simulink model "IntegralBacksteppingDroneControl"  (R2023b)
settings: Solver=VariableStepAuto  StartTime=0.0  StopTime=10.0  RelTol=1e-3
libraries: simulink x1
settings Model: Creator=kevin  LastModifiedBy=kevin

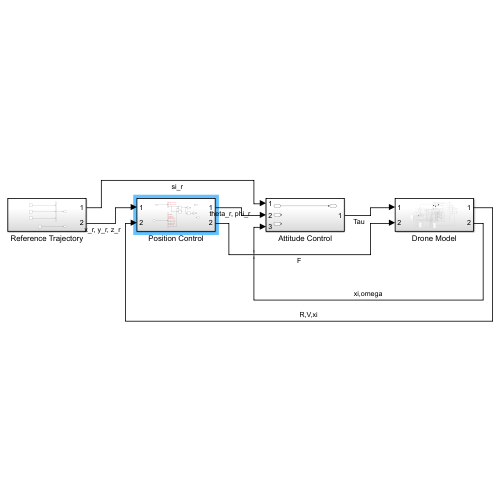
[thumbnail: Simulink's stored preview of the top-level diagram]
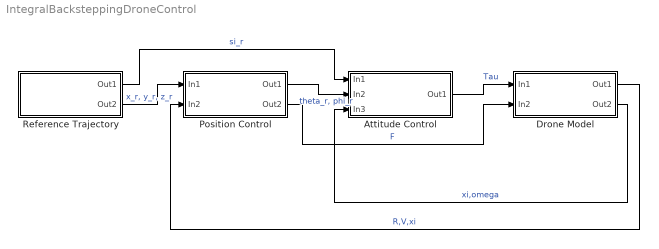
== system IntegralBacksteppingDroneControl ==
  Attitude Control : Subsystem
  Drone Model : Subsystem
  Position Control : Subsystem
  Reference Trajectory : Subsystem
  wires:
  Reference Trajectory/2(Out2) -> Position Control/1(In1)  "x_r, y_r, z_r"
  Reference Trajectory/1(Out1) -> Attitude Control/1(In1)  "si_r"
  Drone Model/1(Out1) -> Position Control/2(In2)  "R,V,xi"
  Drone Model/2(Out2) -> Attitude Control/3(In3)  "xi,omega"
  Position Control/1(Out1) -> Attitude Control/2(In2)  "theta_r, phi_r"
  Position Control/2(Out2) -> Drone Model/2(In2)  "F"
  Attitude Control/1(Out1) -> Drone Model/1(In1)  "Tau"

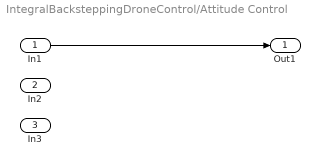
== system IntegralBacksteppingDroneControl/Attitude Control ==
  In1 : Inport
  In2 : Inport  Port=2
  In3 : Inport  Port=3
  Out1 : Outport
  wires:
  In1/1 -> Out1/1

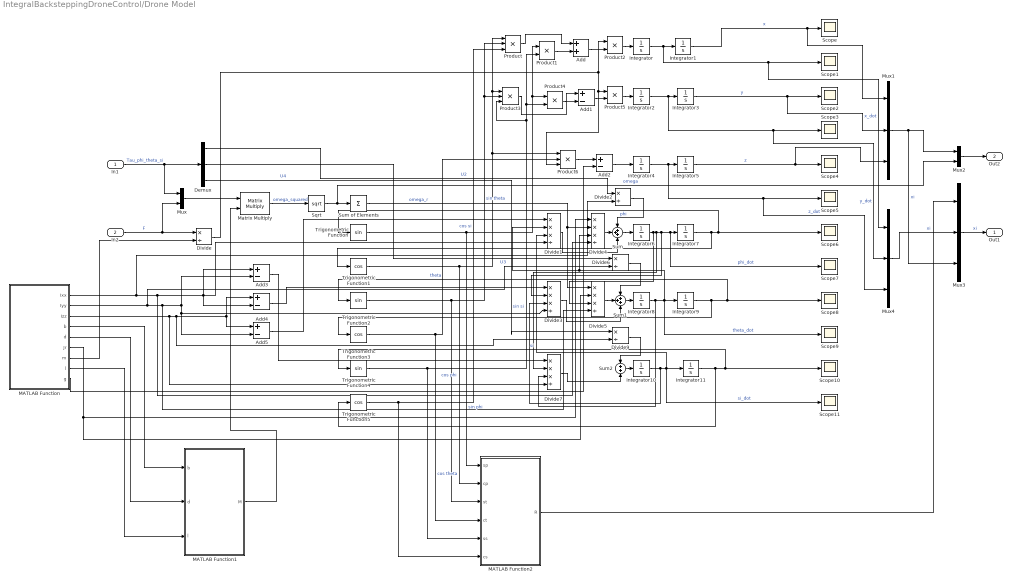
== system IntegralBacksteppingDroneControl/Drone Model ==
  In1 : Inport
  In2 : Inport  Port=2
  Add : Sum
  Add{1..5} (5 alike) : Sum  Inputs=+-
  Demux : Demux  Outputs=3
  Divide{,2,6,9} (4 alike) : Product  Inputs=*/
  Divide{1,3..5,7} (5 alike) : Product  Inputs=***/
  Integrator{,1..11} (12 alike) : Integrator
  MATLAB Function : MATLAB Function  TreatAsAtomicUnit=on
  MATLAB Function1 : MATLAB Function  TreatAsAtomicUnit=on
  MATLAB Function2 : MATLAB Function  TreatAsAtomicUnit=on
  Matrix Multiply : Product  Multiplication=Matrix(*)
  Mux : Mux  Inputs=2
  Mux1 : Mux  Inputs=3
  Mux2 : Mux  Inputs=2
  Mux3 : Mux  Inputs=3
  Mux4 : Mux  Inputs=3
  Product : Product  Inputs=3
  Product{1..2,4..5} (4 alike) : Product
  Product3 : Product  Inputs=3
  Product6 : Product  Inputs=3
  Scope{,1..11} (12 alike) : Scope
  Sqrt : Sqrt
  Sum : Sum  Inputs=+++
  Sum of Elements : Sum  Inputs=+
  Sum1 : Sum  Inputs=+++
  Sum2 : Sum
  Trigonometric Function : Trigonometry
  Trigonometric Function1 : Trigonometry  Operator=cos
  Trigonometric Function2 : Trigonometry
  Trigonometric Function3 : Trigonometry  Operator=cos
  Trigonometric Function4 : Trigonometry
  Trigonometric Function5 : Trigonometry  Operator=cos
  Out1 : Outport
  Out2 : Outport  Port=2
  wires:
  In1/1 -> Demux/1, Mux/1  "Tau_phi_theta_si"
  In2/1 -> Mux/2, Divide/1  "F"
  Demux/1 -> Divide2/1  "U2"
  Demux/2 -> Divide6/1  "U3"
  Demux/3 -> Divide9/1  "U4"
  Integrator1/1 -> Mux1/1, Scope/1  "x"
  Integrator/1 -> Mux4/1, Scope1/1, Integrator1/1  "x_dot"
  Integrator3/1 -> Mux1/2, Scope2/1  "y"
  Integrator2/1 -> Mux4/2, Scope3/1, Integrator3/1  "y_dot"
  Integrator5/1 -> Mux1/3, Scope4/1  "z"
  Integrator4/1 -> Mux4/3, Scope5/1, Integrator5/1  "z_dot"
  Integrator7/1 -> Trigonometric Function1/1, Trigonometric Function/1, Scope6/1  "phi"
  Integrator6/1 -> Divide5/3, Scope7/1, Integrator7/1, Divide3/2, Divide7/2  "phi_dot"
  Integrator9/1 -> Trigonometric Function3/1, Trigonometric Function2/1, Scope8/1  "theta"
  Integrator8/1 -> Divide7/3, Divide1/2, Divide4/3, Scope9/1, Integrator9/1  "theta_dot"
  Integrator11/1 -> Trigonometric Function5/1, Trigonometric Function4/1, Scope10/1  "si"
  Integrator10/1 -> Divide3/3, Divide1/3, Scope11/1, Integrator11/1  "si_dot"
  Trigonometric Function/1 -> MATLAB Function2/1(sp), Product1/1, Product4/1  "sin phi"
  Trigonometric Function1/1 -> MATLAB Function2/2(cp), Product3/1, Product/1, Product6/1  "cos phi"
  Trigonometric Function2/1 -> MATLAB Function2/3(st), Product3/2, Product/2  "sin theta"
  Trigonometric Function3/1 -> MATLAB Function2/4(ct), Product6/2  "cos theta"
  Trigonometric Function4/1 -> MATLAB Function2/5(ss), Product3/3, Product1/2, Product4/2  "sin si"
  Trigonometric Function5/1 -> MATLAB Function2/6(cs), Product/3  "cos si"
  Product/1 -> Add/1
  Product1/1 -> Add/2
  MATLAB Function/7(m) -> Divide/2
  Divide/1 -> Product2/1, Product6/3, Product5/1
  Product2/1 -> Integrator/1
  Add/1 -> Product2/2
  Product3/1 -> Add1/1
  Product4/1 -> Add1/2
  Product5/1 -> Integrator2/1
  Add1/1 -> Product5/2
  Product6/1 -> Add2/1
  MATLAB Function/9(g) -> Add2/2
  Add2/1 -> Integrator4/1
  MATLAB Function/4(b) -> MATLAB Function1/1(b)
  MATLAB Function/8(l) -> MATLAB Function1/3(l)
  MATLAB Function1/1(M) -> Matrix Multiply/2
  Mux/1 -> Matrix Multiply/1
  Matrix Multiply/1 -> Sqrt/1  "omega_squared"
  Sqrt/1 -> Mux2/2, Sum of Elements/1  "omega"
  Sum of Elements/1 -> Divide5/1, Divide4/2  "omega_r"
  Add3/1 -> Divide7/1
  Add4/1 -> Divide3/1
  Add5/1 -> Divide1/1
  Divide1/1 -> Sum/3
  MATLAB Function/5(d) -> MATLAB Function1/2(d)
  MATLAB Function/1(Ixx) -> Divide2/2, Divide4/4, Divide1/4, Add3/1, Add4/2
  Divide4/1 -> Sum/2
  Sum/1 -> Integrator6/1
  Divide2/1 -> Sum/1
  Sum1/1 -> Integrator8/1
  Divide5/1 -> Sum1/2
  Divide3/1 -> Sum1/3
  Divide6/1 -> Sum1/1
  MATLAB Function/6(Jr) -> Divide4/1, Divide5/2
  MATLAB Function/2(Iyy) -> Divide6/2, Divide5/4, Divide3/4, Add5/2, Add3/2
  Sum2/1 -> Integrator10/1
  Divide7/1 -> Sum2/2
  Divide9/1 -> Sum2/1
  MATLAB Function/3(Izz) -> Divide7/4, Divide9/2, Add5/1, Add4/1
  Mux1/1 -> Mux3/3, Mux2/1  "xi"
  Mux2/1 -> Out2/1
  MATLAB Function2/1(R) -> Mux3/1
  Mux3/1 -> Out1/1  "xi"
  Mux4/1 -> Mux3/2  "xi"

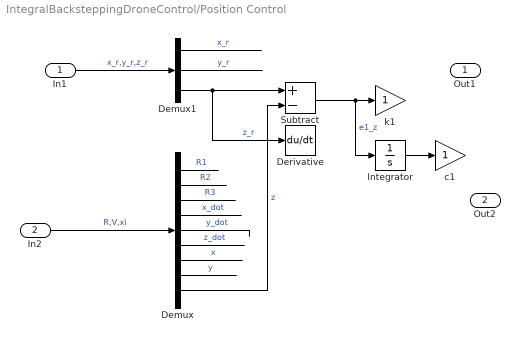
== system IntegralBacksteppingDroneControl/Position Control ==
  In1 : Inport
  In2 : Inport  Port=2
  Demux : Demux  Outputs=9
  Demux1 : Demux  Outputs=3
  Derivative : Derivative
  Integrator : Integrator
  Subtract : Sum  Inputs=+-
  c1 : Gain
  k1 : Gain
  Out1 : Outport
  Out2 : Outport  Port=2
  wires:
  In1/1 -> Demux1/1  "x_r,y_r,z_r"
  In2/1 -> Demux/1  "R,V,xi"
  Demux/1 -> ?  "R1"
  Demux/2 -> ?  "R2"
  Demux/3 -> ?  "R3"
  Demux/4 -> ?  "x_dot"
  Demux/5 -> ?  "y_dot"
  Demux/6 -> ?  "z_dot"
  Demux/7 -> ?  "x"
  Demux/8 -> ?  "y"
  Demux/9 -> Subtract/2  "z"
  Demux1/1 -> ?  "x_r"
  Demux1/2 -> ?  "y_r"
  Demux1/3 -> Derivative/1, Subtract/1  "z_r"
  Subtract/1 -> Integrator/1, k1/1  "e1_z"
  Integrator/1 -> c1/1

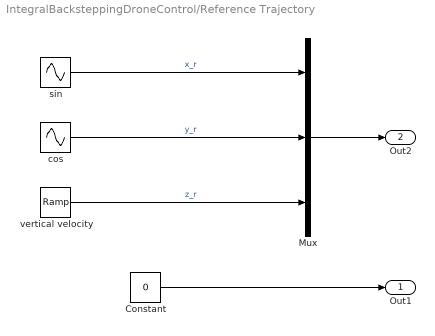
== system IntegralBacksteppingDroneControl/Reference Trajectory ==
  Constant : Constant  Value=0
  Mux : Mux  Inputs=3
  cos : Sin  Amplitude=2  Frequency=0.1*pi  Phase=pi/2  SampleTime=0.001
  sin : Sin  Amplitude=2  Frequency=0.1*pi  SampleTime=0.001
  vertical velocity : simulink/Sources/Ramp  slope=0.2  start=0  InitialOutput=0
  Out1 : Outport
  Out2 : Outport  Port=2
  wires:
  sin/1 -> Mux/1  "x_r"
  cos/1 -> Mux/2  "y_r"
  vertical velocity/1 -> Mux/3  "z_r"
  Mux/1 -> Out2/1
  Constant/1 -> Out1/1

== matlab function IntegralBacksteppingDroneControl/Drone Model/MATLAB Function1 ==
  data: M output; b input; d input; l input
function M  = fcn(b, d, l)
    %% Parameters %%
    M = inv([b, b, b, b;
        0, -b*l, 0, b*l;
        -b*l 0 b*l 0;
        d; -d; d; -d]);
end

== matlab function IntegralBacksteppingDroneControl/Drone Model/MATLAB Function ==
  data: Ixx output; Iyy output; Izz output; b output; d output; Jr output; m output; l output; g output
function [Ixx, Iyy, Izz, b, d, Jr, m, l, g] = fcn()
%% Parameters %%
Ixx = 4.856e-3;
Iyy = 4.856e-3;
Izz = 8.801e-3;
b = 2.980e-6;
d = 1.140e-7;
Jr = (0.004/3)*((5/2)*0.0254)^2;
m = 0.468;
l = 0.225;
g = 9.81;

== matlab function IntegralBacksteppingDroneControl/Drone Model/MATLAB Function2 ==
  data: R output; sp input; cp input; st input; ct input; ss input; cs input
function R = fcn(sp,cp,st,ct,ss,cs)
    R = [cs*ct, sp*st*cs - cp*ss, cp*st*cs + sp*ss; 
        ss*ct, sp*st*ss + cp*cs, cp*st*ss-sp*cs; 
        -st, sp*ct, cp*ct];
end
